simulink model "project2"  (R2023b)
settings: Solver=VariableStepAuto  StartTime=0.0  StopTime=10.0  RelTol=1e-3
values from neighbouring files (symbols this model uses):
  c_alphaf = 1    [MEEN432_Project2_init.m]
  c_alphar = 1    [MEEN432_Project2_init.m]
  L = lf + lr    (= 4)    [MEEN432_Project2_init.m]
  lf = 2    [MEEN432_Project2_init.m]
  lr = 2    [MEEN432_Project2_init.m]
  R = 200    [MEEN432_Project2_init.m]
undefined symbols (not defined in the file or in its folder): vxd
settings Model: Creator=flare  LastModifiedBy=flare

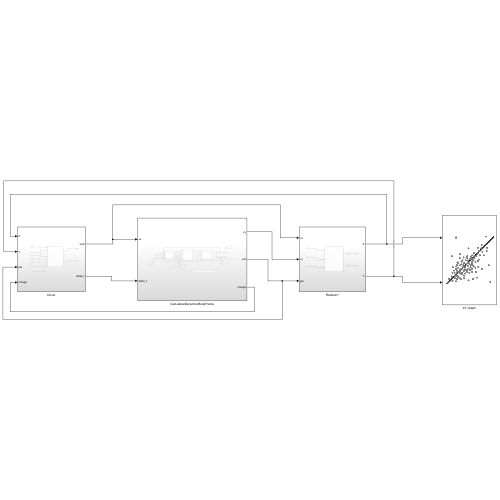
[thumbnail: Simulink's stored preview of the top-level diagram]
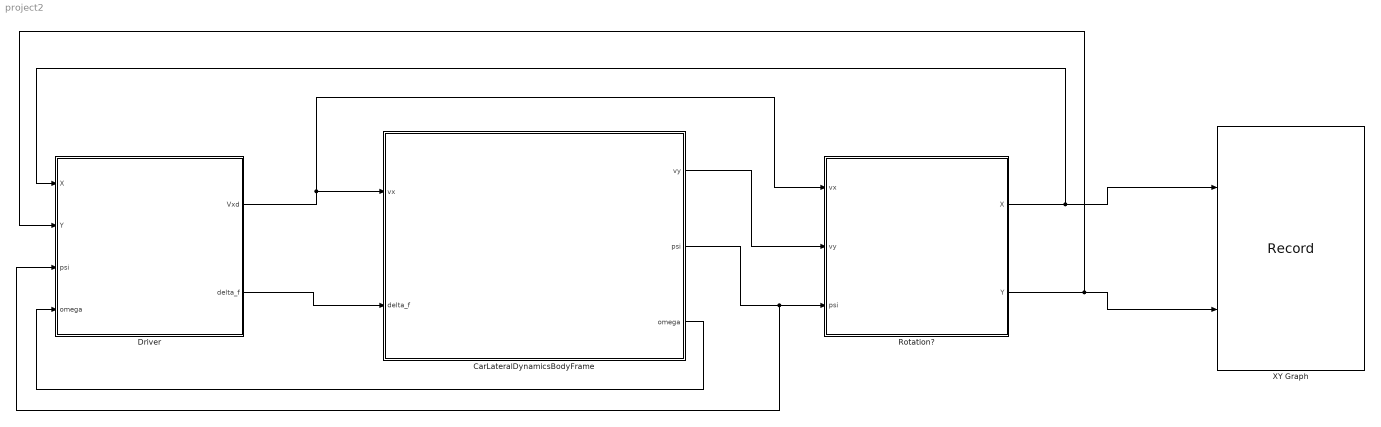
== system project2 ==
  CarLateralDynamicsBodyFrame : Subsystem
  Driver : Subsystem
  Rotation? : Subsystem
  XY Graph : Record  FileSettingsInternal="{\"entries\":[{\"content\":{\"excelSettings\":{\"content\":{},\"type\":\"Streamout.ExcelSettings\"}},\"type\":\"Streamout.FileSettingStorage\",\"uuid\":\"\"}],\"packageUris\":[\"http:\\/\\/schema.mathworks.com\\/mf0\\/streamout_blocks\\/R2020a\"],\"version\":\"1.0\"}"  Layout=[1 1]  SignalsInternal="{\"entries\":[{\"content\":{\"signals\":[{\"content\":{\"blockPath\":[],\"dimensions\":[1],\"domain\":\"\",\"lineColor\":\"#a2142f\",\"plots\":[1],\"port\":1,\"sid\":[\"\"],\"signalID\":206,\"signalName\":\"Rotation?:1\"},\"type\":\"RecordBlkView.Signal\",\"uuid\":\"\"},{\"content\":{\"blockPath\":[],\"dimensions\":[1],\"domain\":\"\",\"lineColor\":\"#139fff\",\"plots\":[1],\"port\":2,\"sid\":[\"\"],\"signalID\":210,\"signalName\":\"Rotation?:2\"},\"type\":\"RecordBlkView.Signal\",\"uuid\":\"\"}]},\"type\":\"RecordBlkView.InputSignals\",\"uuid\":\"\"}],\"packageUris\":[\"http:\\/\\/schema.mathworks.com\\/mf0\\/streamout_blocks\\/R2020a\"],\"version\":\"1.0\"}"  VisualizationBindings="{\"xyplotplugin\":{\"info\":[{\"series\":[{\"bindingParametersList\":[{\"parameter\":\"X-Axis\",\"signalID\":206,\"signalName\":\"Rotation?:1\"},{\"parameter\":\"Y-Axis\",\"signalID\":210,\"signalName\":\"Rotation?:2\"}],\"seriesID\":27384}],\"subplotID\":1}]}}"  CompatibilityTag=XY
  wires:
  Rotation?/1(X) -> Driver/1(X), XY Graph/1
  Rotation?/2(Y) -> Driver/2(Y), XY Graph/2
  Driver/1(Vxd) -> Rotation?/1(vx), CarLateralDynamicsBodyFrame/1(vx)
  Driver/2(delta_f) -> CarLateralDynamicsBodyFrame/2(delta_f)
  CarLateralDynamicsBodyFrame/1(vy) -> Rotation?/2(vy)
  CarLateralDynamicsBodyFrame/2(psi) -> Driver/3(psi), Rotation?/3(psi)
  CarLateralDynamicsBodyFrame/3(omega) -> Driver/4(omega)

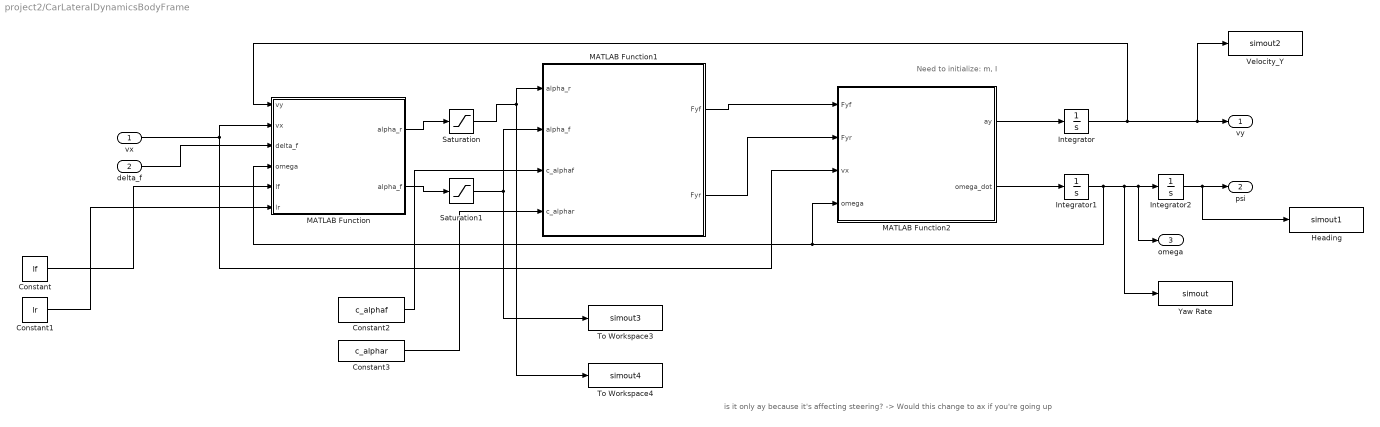
== system project2/CarLateralDynamicsBodyFrame ==
  note: is it only ay because it's affecting steering? -> Would this change to ax if you're going up
  note: Need to initialize: m, I
  vx : Inport
  delta_f : Inport  Port=2
  Constant : Constant  Value=lf
  Constant1 : Constant  Value=lr
  Constant2 : Constant  Value=c_alphaf
  Constant3 : Constant  Value=c_alphar
  Heading : ToWorkspace  VariableName=simout1  SaveFormat=Timeseries  SampleTime=-1
  Integrator : Integrator
  Integrator1 : Integrator
  Integrator2 : Integrator
  MATLAB Function : MATLAB Function  TreatAsAtomicUnit=on
  MATLAB Function1 : MATLAB Function  TreatAsAtomicUnit=on
  MATLAB Function2 : MATLAB Function  TreatAsAtomicUnit=on
  Saturation : Saturate
  Saturation1 : Saturate
  To Workspace3 : ToWorkspace  VariableName=simout3  SaveFormat=Timeseries  SampleTime=-1
  To Workspace4 : ToWorkspace  VariableName=simout4  SaveFormat=Timeseries  SampleTime=-1
  Velocity_Y : ToWorkspace  VariableName=simout2  SaveFormat=Timeseries  SampleTime=-1
  Yaw Rate : ToWorkspace  VariableName=simout  SaveFormat=Timeseries  SampleTime=-1
  vy : Outport
  psi : Outport  Port=2
  omega : Outport  Port=3
  wires:
  MATLAB Function/1(alpha_r) -> Saturation/1
  MATLAB Function/2(alpha_f) -> Saturation1/1
  MATLAB Function2/2(omega_dot) -> Integrator1/1
  MATLAB Function2/1(ay) -> Integrator/1
  Integrator1/1 -> MATLAB Function2/4(omega), MATLAB Function/4(omega), Yaw Rate/1, omega/1, Integrator2/1
  Integrator/1 -> MATLAB Function/1(vy), Velocity_Y/1, vy/1
  Integrator2/1 -> Heading/1, psi/1
  vx/1 -> MATLAB Function2/3(vx), MATLAB Function/2(vx)
  delta_f/1 -> MATLAB Function/3(delta_f)
  Saturation/1 -> To Workspace4/1, MATLAB Function1/1(alpha_r)
  Saturation1/1 -> To Workspace3/1, MATLAB Function1/2(alpha_f)
  MATLAB Function1/1(Fyf) -> MATLAB Function2/1(Fyf)
  MATLAB Function1/2(Fyr) -> MATLAB Function2/2(Fyr)
  Constant/1 -> MATLAB Function/5(lf)
  Constant1/1 -> MATLAB Function/6(lr)
  Constant2/1 -> MATLAB Function1/3(c_alphaf)
  Constant3/1 -> MATLAB Function1/4(c_alphar)

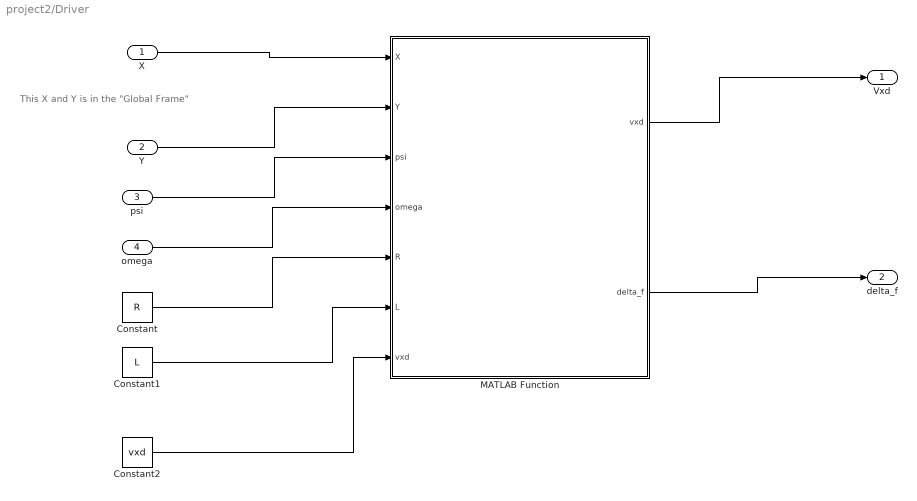
== system project2/Driver ==
  note: This X and Y is in the "Global Frame"
  X : Inport
  Y : Inport  Port=2
  psi : Inport  Port=3
  omega : Inport  Port=4
  Constant : Constant  Value=R
  Constant1 : Constant  Value=L
  Constant2 : Constant  Value=vxd
  MATLAB Function : MATLAB Function  TreatAsAtomicUnit=on
  Vxd : Outport
  delta_f : Outport  Port=2
  wires:
  Y/1 -> MATLAB Function/2(Y)
  psi/1 -> MATLAB Function/3(psi)
  omega/1 -> MATLAB Function/4(omega)
  MATLAB Function/1(vxd) -> Vxd/1
  MATLAB Function/2(delta_f) -> delta_f/1
  X/1 -> MATLAB Function/1(X)
  Constant/1 -> MATLAB Function/5(R)
  Constant1/1 -> MATLAB Function/6(L)
  Constant2/1 -> MATLAB Function/7("vxd ")

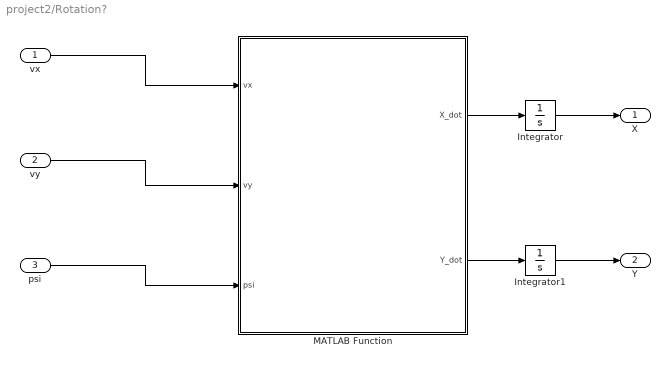
== system project2/Rotation? ==
  vx : Inport
  vy : Inport  Port=2
  psi : Inport  Port=3
  Integrator : Integrator
  Integrator1 : Integrator
  MATLAB Function : MATLAB Function  TreatAsAtomicUnit=on
  X : Outport
  Y : Outport  Port=2
  wires:
  vx/1 -> MATLAB Function/1(vx)
  vy/1 -> MATLAB Function/2(vy)
  MATLAB Function/1(X_dot) -> Integrator/1
  MATLAB Function/2(Y_dot) -> Integrator1/1
  Integrator/1 -> X/1
  Integrator1/1 -> Y/1
  psi/1 -> MATLAB Function/3(psi)

== matlab function project2/CarLateralDynamicsBodyFrame/MATLAB Function ==
  data: vy input; alpha_r output; vx input; delta_f input; omega input; alpha_f output; lf input; lr input
function [alpha_r, alpha_f] = fcn(vy, vx, delta_f, omega, lf, lr)

alpha_f = delta_f - atan((vy+lf*omega)/vx);
alpha_r = atan((vy-lr*omega)/vx);

== matlab function project2/Driver/MATLAB Function ==
  data: X input; Y input; psi input; omega input; vxd output; delta_f output; R input; L input; vxd input
function [vxd, delta_f] = fcn(X, Y, psi, omega, R, L, vxd)

vx = omega*R;
delta_f = L*omega/vx;

== matlab function project2/CarLateralDynamicsBodyFrame/MATLAB Function1 ==
  data: alpha_r input; Fyf output; alpha_f input; Fyr output; c_alphaf input; c_alphar input
function [Fyf, Fyr] = fcn(alpha_r, alpha_f, c_alphaf, c_alphar)

Fyf = c_alphaf * alpha_r;
Fyr = c_alphar * alpha_f;

== matlab function project2/CarLateralDynamicsBodyFrame/MATLAB Function2 ==
  data: Fyf input; ay output; Fyr input; vx input; omega input; omega_dot output
function [ay, omega_dot] = fcn(Fyf, Fyr, vx, omega)

ay= vx*omega + (Fyf+Fyr); %/m;
omega_dot = (Fyf - Fyr);  %/I;

== matlab function project2/Rotation?/MATLAB Function ==
  data: vx input; X_dot output; vy input; psi input; Y_dot output
function [X_dot, Y_dot] = fcn(vx, vy, psi)


rot = [cos(psi) -sin(psi) ; sin(psi) cos(psi)];
v = [vx;vy];

temp = rot * v;

X_dot = temp(1);
Y_dot = temp(2);
